simulink model "APF_Path_Planning_2023a"  (R2023a)
settings: Solver=ode4  StartTime=0.0  StopTime=tsim  FixedStep=baseRate  RelTol=1e-6  AbsTol=1e-6
values from neighbouring files (symbols this model uses):
  A = [0 0 0 1 0 0 ... (first row only)    [CTL.m]
  a = 25.028    [CTL.m]
  a1 = gain_matrix(1,1)    [CTL.m]
  alpha_m = 0.1    [CTL.m]
  alphap = 1    [CTL.m]
  alphat = 1.1    [CTL.m]
  Am = [0 0 1 0; 0 0 0 1; -wn^2 0 -2*zeta*wn 0; 0 -wn^2 0 -2*zeta*wn]    [CTL.m]
  b = gain_matrix(1,2)    [CTL.m]
  Bm = [0 0; 0 0; -wn^2 0; 0 -wn^2]    [CTL.m]
  c = gain_matrix(2,1)    [CTL.m]
  Cm = [alpha_m 0 0 0; 0 alpha_m 0 0; 0 0 1 0; 0 0 0 1]    [CTL.m]
  d = gain_matrix(2,2)    [CTL.m]
  Dm = zeros(4,2)    [CTL.m]
  epsilon = F_max/2    (= 0.11)    [CTL.m]
  F_max = 0.22    [CTL.m]
  Hz = 0.01    [CTL.m]
  J = IRED    [CTL.m]
  k = lqr(A,B1,Q,R)    [CTL.m]
  k1 = 5    [CTL.m]
  k1t = 2    [CTL.m]
  k2 = 28    [CTL.m]
  k2t = 16    [CTL.m]
  k_1_0 = 3.5    [CTL.m]
  k_1_t_0 = 1    [CTL.m]
  k_2_0 = 28    [CTL.m]
  k_2_t_0 = 1    [CTL.m]
  Kd_t = 9.5    [CTL.m]
  Kd_x = 28    [CTL.m]
  Kd_y = Kd_x    (= 28)    [CTL.m]
  Kp_t = 1    [CTL.m]
  Kp_x = 3.5    [CTL.m]
  Kp_y = Kp_x    (= 3.5)    [CTL.m]
  lambda1 = 0.4    [CTL.m]
  lambda12 = 0.4    [CTL.m]
  lambda12_t = 0.05    [CTL.m]
  lambda1_t = 0.05    [CTL.m]
  lambda2 = 0.4    [CTL.m]
  lambda2_t = 0.05    [CTL.m]
  m = mRED    [CTL.m]
  p = 0.4    [CTL.m]
  p_t = 0.05    [CTL.m]
  Q = [w 0 0 0 0 0 ... (first row only)    [CTL.m]
  R = [r 0 0 ... (first row only)    [CTL.m]
  Red_Rate = 0.025    [CTL.m]
  T_max = 0.0235    [CTL.m]
  Time_Look = 25    [CTL.m]
  xm_0 = [RED_ini(1,1:2),0,0]    [CTL.m]
undefined symbols (not defined in the file or in its folder): a2, a3, adadelta_epsilon, adadelta_gamma, adagrad_epsilon, adagrad_eta, adam_beta_1, adam_beta_2, adam_epsilon, adam_eta, adamax_beta_1, adamax_beta_2, adamax_eta, alpha, Att_Mode, b0, b1, b2, b3, baseRate, beta, Binv, BLACK_end, BLACK_ini, BLUE_end, BLUE_ini, DiscIntNeverNeededParam, drop_states_ARM, drop_states_BLACK, drop_states_BLUE, drop_states_RED, dt, end_time_black, end_time_blue, F_Black_X_nominal, F_Black_Y_nominal, F_Blue_X_nominal, F_Blue_Y_nominal, F_red_X_nominal, F_red_Y_nominal, F_thrusters_BLACK, F_thrusters_BLUE, F_thrusters_RED, Gamma1_el, Gamma1_sh, Gamma1_wr, Gamma2_el, Gamma2_sh, Gamma2_wr, Gamma3_el, Gamma3_sh, Gamma3_wr, Gamma4_el, Gamma4_sh, Gamma4_wr, Gamma5_el, Gamma5_sh, Gamma5_wr, Gamma6_el, Gamma6_sh ... (+98)
libraries: nvidiaSharedBlocks x10, MainLibrary x4, dspsigops x4, simulink x2, etargetslib x1
(part 11 of 13)

== system APF_Path_Planning_2023a/Phase #3: Experiment/Change RED Behavior/Sub-Phase #4/RED+ARM/Simulated Position Controller/Custom Discrete PD (Elbow)/x_dot -> x2 ==
  note: dy/dt ~= (y2-y1)/deltaT
  y(t) : Inport
  Delay1 : Delay  DelayLength=1  InitialConditionSource=Input port
      settings: InputPortMap=u0,p4
  Hold this value : Subsystem  TreatAsAtomicUnit=on
  Sum6 : Sum  Inputs=-+|
  divide by delta T : Gain  Gain=1/baseRate
  "if we went through a \"step\"" : If  IfExpression=u1 ~= 0  ShowElse=off
  dy(t)/dt : Outport  VectorParamsAs1DForOutWhenUnconnected=off
  wires:
  divide by delta T/1 -> dy(t)/dt/1
  Delay1/1 -> Sum6/1
  "if we went through a \"step\""/1 -> Hold this value/Action
  Hold this value/1(Out1) -> divide by delta T/1
  Sum6/1 -> "if we went through a \"step\""/1, Hold this value/1(In1)
  y(t)/1 -> Sum6/2, Delay1/2, Delay1/1

== system APF_Path_Planning_2023a/Phase #3: Experiment/Change RED Behavior/Sub-Phase #4/RED+ARM/Simulated Position Controller/Custom Discrete PD (Shoulder)/x_dot -> x2 ==
  note: dy/dt ~= (y2-y1)/deltaT
  y(t) : Inport
  Delay1 : Delay  DelayLength=1  InitialConditionSource=Input port
      settings: InputPortMap=u0,p4
  Hold this value : Subsystem  TreatAsAtomicUnit=on
  Sum6 : Sum  Inputs=-+|
  divide by delta T : Gain  Gain=1/baseRate
  "if we went through a \"step\"" : If  IfExpression=u1 ~= 0  ShowElse=off
  dy(t)/dt : Outport  VectorParamsAs1DForOutWhenUnconnected=off
  wires:
  divide by delta T/1 -> dy(t)/dt/1
  Delay1/1 -> Sum6/1
  "if we went through a \"step\""/1 -> Hold this value/Action
  Hold this value/1(Out1) -> divide by delta T/1
  Sum6/1 -> "if we went through a \"step\""/1, Hold this value/1(In1)
  y(t)/1 -> Sum6/2, Delay1/2, Delay1/1

== system APF_Path_Planning_2023a/Phase #3: Experiment/Change RED Behavior/Sub-Phase #4/RED+ARM/Simulated Position Controller/Custom Discrete PD (Wrist)/x_dot -> x2 ==
  note: dy/dt ~= (y2-y1)/deltaT
  y(t) : Inport
  Delay1 : Delay  DelayLength=1  InitialConditionSource=Input port
      settings: InputPortMap=u0,p4
  Hold this value : Subsystem  TreatAsAtomicUnit=on
  Sum6 : Sum  Inputs=-+|
  divide by delta T : Gain  Gain=1/baseRate
  "if we went through a \"step\"" : If  IfExpression=u1 ~= 0  ShowElse=off
  dy(t)/dt : Outport  VectorParamsAs1DForOutWhenUnconnected=off
  wires:
  divide by delta T/1 -> dy(t)/dt/1
  Delay1/1 -> Sum6/1
  "if we went through a \"step\""/1 -> Hold this value/Action
  Hold this value/1(Out1) -> divide by delta T/1
  Sum6/1 -> "if we went through a \"step\""/1, Hold this value/1(In1)
  y(t)/1 -> Sum6/2, Delay1/2, Delay1/1

== system APF_Path_Planning_2023a/Phase #4: Return Home/Change RED Behavior/RED+ARM/Simulated Position Controller/Custom Discrete PD (Elbow)/x_dot -> x2/Hold this value ==
  In1 : Inport
  Action Port : ActionPort  ActionPortLabel=if(u1 ~= 0)
  Out1 : Outport  VectorParamsAs1DForOutWhenUnconnected=off
  wires:
  In1/1 -> Out1/1

== system APF_Path_Planning_2023a/Phase #4: Return Home/Change RED Behavior/RED+ARM/Simulated Position Controller/Custom Discrete PD (Shoulder)/x_dot -> x2/Hold this value ==
  In1 : Inport
  Action Port : ActionPort  ActionPortLabel=if(u1 ~= 0)
  Out1 : Outport  VectorParamsAs1DForOutWhenUnconnected=off
  wires:
  In1/1 -> Out1/1

== system APF_Path_Planning_2023a/Phase #4: Return Home/Change RED Behavior/RED+ARM/Simulated Position Controller/Custom Discrete PD (Wrist)/x_dot -> x2/Hold this value ==
  In1 : Inport
  Action Port : ActionPort  ActionPortLabel=if(u1 ~= 0)
  Out1 : Outport  VectorParamsAs1DForOutWhenUnconnected=off
  wires:
  In1/1 -> Out1/1

== system APF_Path_Planning_2023a/Phase #5: Hold Home/Change RED Behavior/RED+ARM/Simulated Position Controller/Custom Discrete PD (Elbow)/x_dot -> x2/Hold this value ==
  In1 : Inport
  Action Port : ActionPort  ActionPortLabel=if(u1 ~= 0)
  Out1 : Outport  VectorParamsAs1DForOutWhenUnconnected=off
  wires:
  In1/1 -> Out1/1

== system APF_Path_Planning_2023a/Phase #5: Hold Home/Change RED Behavior/RED+ARM/Simulated Position Controller/Custom Discrete PD (Shoulder)/x_dot -> x2/Hold this value ==
  In1 : Inport
  Action Port : ActionPort  ActionPortLabel=if(u1 ~= 0)
  Out1 : Outport  VectorParamsAs1DForOutWhenUnconnected=off
  wires:
  In1/1 -> Out1/1

== system APF_Path_Planning_2023a/Phase #5: Hold Home/Change RED Behavior/RED+ARM/Simulated Position Controller/Custom Discrete PD (Wrist)/x_dot -> x2/Hold this value ==
  In1 : Inport
  Action Port : ActionPort  ActionPortLabel=if(u1 ~= 0)
  Out1 : Outport  VectorParamsAs1DForOutWhenUnconnected=off
  wires:
  In1/1 -> Out1/1

== system APF_Path_Planning_2023a/Phase #3: Experiment/Change RED Behavior/Sub-Phase #1/RED+ARM/Simulated Position Controller/Custom Discrete PD (Elbow)/x_dot -> x2/Hold this value ==
  In1 : Inport
  Action Port : ActionPort  ActionPortLabel=if(u1 ~= 0)
  Out1 : Outport  VectorParamsAs1DForOutWhenUnconnected=off
  wires:
  In1/1 -> Out1/1

== system APF_Path_Planning_2023a/Phase #3: Experiment/Change RED Behavior/Sub-Phase #1/RED+ARM/Simulated Position Controller/Custom Discrete PD (Shoulder)/x_dot -> x2/Hold this value ==
  In1 : Inport
  Action Port : ActionPort  ActionPortLabel=if(u1 ~= 0)
  Out1 : Outport  VectorParamsAs1DForOutWhenUnconnected=off
  wires:
  In1/1 -> Out1/1

== system APF_Path_Planning_2023a/Phase #3: Experiment/Change RED Behavior/Sub-Phase #1/RED+ARM/Simulated Position Controller/Custom Discrete PD (Wrist)/x_dot -> x2/Hold this value ==
  In1 : Inport
  Action Port : ActionPort  ActionPortLabel=if(u1 ~= 0)
  Out1 : Outport  VectorParamsAs1DForOutWhenUnconnected=off
  wires:
  In1/1 -> Out1/1

== system APF_Path_Planning_2023a/Phase #3: Experiment/Change RED Behavior/Sub-Phase #2 /RED+ARM/Simulated Position Controller/Custom Discrete PD (Elbow)/x_dot -> x2/Hold this value ==
  In1 : Inport
  Action Port : ActionPort  ActionPortLabel=if(u1 ~= 0)
  Out1 : Outport  VectorParamsAs1DForOutWhenUnconnected=off
  wires:
  In1/1 -> Out1/1

== system APF_Path_Planning_2023a/Phase #3: Experiment/Change RED Behavior/Sub-Phase #2 /RED+ARM/Simulated Position Controller/Custom Discrete PD (Shoulder)/x_dot -> x2/Hold this value ==
  In1 : Inport
  Action Port : ActionPort  ActionPortLabel=if(u1 ~= 0)
  Out1 : Outport  VectorParamsAs1DForOutWhenUnconnected=off
  wires:
  In1/1 -> Out1/1

== system APF_Path_Planning_2023a/Phase #3: Experiment/Change RED Behavior/Sub-Phase #2 /RED+ARM/Simulated Position Controller/Custom Discrete PD (Wrist)/x_dot -> x2/Hold this value ==
  In1 : Inport
  Action Port : ActionPort  ActionPortLabel=if(u1 ~= 0)
  Out1 : Outport  VectorParamsAs1DForOutWhenUnconnected=off
  wires:
  In1/1 -> Out1/1

== system APF_Path_Planning_2023a/Phase #3: Experiment/Change RED Behavior/Sub-Phase #3 /RED+ARM/Simulated Position Controller/Custom Discrete PD (Elbow)/x_dot -> x2/Hold this value ==
  In1 : Inport
  Action Port : ActionPort  ActionPortLabel=if(u1 ~= 0)
  Out1 : Outport  VectorParamsAs1DForOutWhenUnconnected=off
  wires:
  In1/1 -> Out1/1

== system APF_Path_Planning_2023a/Phase #3: Experiment/Change RED Behavior/Sub-Phase #3 /RED+ARM/Simulated Position Controller/Custom Discrete PD (Shoulder)/x_dot -> x2/Hold this value ==
  In1 : Inport
  Action Port : ActionPort  ActionPortLabel=if(u1 ~= 0)
  Out1 : Outport  VectorParamsAs1DForOutWhenUnconnected=off
  wires:
  In1/1 -> Out1/1

== system APF_Path_Planning_2023a/Phase #3: Experiment/Change RED Behavior/Sub-Phase #3 /RED+ARM/Simulated Position Controller/Custom Discrete PD (Wrist)/x_dot -> x2/Hold this value ==
  In1 : Inport
  Action Port : ActionPort  ActionPortLabel=if(u1 ~= 0)
  Out1 : Outport  VectorParamsAs1DForOutWhenUnconnected=off
  wires:
  In1/1 -> Out1/1

== system APF_Path_Planning_2023a/Phase #3: Experiment/Change RED Behavior/Sub-Phase #4/CTL/Subsystem1/Custom Discrete PD (Attitude)/x_dot -> x2/Hold this value ==
  In1 : Inport
  Action Port : ActionPort  ActionPortLabel=if(u1 ~= 0)
  Out1 : Outport  VectorParamsAs1DForOutWhenUnconnected=off
  wires:
  In1/1 -> Out1/1

== system APF_Path_Planning_2023a/Phase #3: Experiment/Change RED Behavior/Sub-Phase #4/GDC/APF/GDC/Subsystem1/AdaDelta ==
  state_red : Inport
  phi_tot_grad : Inport  Port=2
  Delay : Delay  DelayLength=1  InitialCondition=[0;0;0]
  Delay1 : Delay  DelayLength=1  InitialCondition=[0;0;0]
  MATLAB Function1 : MATLAB Function  TreatAsAtomicUnit=on
  path : Outport
  wires:
  MATLAB Function1/2(Eg) -> Delay/1
  Delay/1 -> MATLAB Function1/3(Eg_old)
  MATLAB Function1/3(Etheta) -> Delay1/1
  Delay1/1 -> MATLAB Function1/4(Etheta_old)
  phi_tot_grad/1 -> MATLAB Function1/2(phi_tot_grad)
  state_red/1 -> MATLAB Function1/1(state_red)
  MATLAB Function1/1(path) -> path/1

== system APF_Path_Planning_2023a/Phase #3: Experiment/Change RED Behavior/Sub-Phase #4/GDC/APF/GDC/Subsystem1/AdaGrad ==
  phit_tot_grad : Inport
  state_red : Inport  Port=2
  Delay3 : Delay  DelayLength=1
  MATLAB Function1 : MATLAB Function  TreatAsAtomicUnit=on
  path : Outport
  wires:
  state_red/1 -> MATLAB Function1/1(state_red)
  Delay3/1 -> MATLAB Function1/3(Gt_old)
  MATLAB Function1/1(path) -> path/1
  phit_tot_grad/1 -> MATLAB Function1/2(phi_tot_grad)
  MATLAB Function1/2(Gt) -> Delay3/1

== system APF_Path_Planning_2023a/Phase #3: Experiment/Change RED Behavior/Sub-Phase #4/GDC/APF/GDC/Subsystem1/AdaMax ==
  phit_tot_grad : Inport
  state_red : Inport  Port=2
  Clock : Clock
  Constant : Constant  Value=Phase2_End
  Delay1 : Delay  DelayLength=1
  Delay3 : Delay  DelayLength=1
  MATLAB Function1 : MATLAB Function  TreatAsAtomicUnit=on
  Sum : Sum  Inputs=|+-
  path : Outport
  wires:
  Delay1/1 -> MATLAB Function1/4(v_old)
  MATLAB Function1/3(v) -> Delay1/1
  MATLAB Function1/2(m) -> Delay3/1
  Delay3/1 -> MATLAB Function1/3(m_old)
  state_red/1 -> MATLAB Function1/1(state_red)
  phit_tot_grad/1 -> MATLAB Function1/2(phi_tot_grad)
  MATLAB Function1/1(path) -> path/1
  Clock/1 -> Sum/1
  Sum/1 -> MATLAB Function1/5(time)
  Constant/1 -> Sum/2

== system APF_Path_Planning_2023a/Phase #3: Experiment/Change RED Behavior/Sub-Phase #4/GDC/APF/GDC/Subsystem1/Adam ==
  phit_tot_grad : Inport
  state_red : Inport  Port=2
  Clock : Clock
  Delay1 : Delay  DelayLength=1
  Delay3 : Delay  DelayLength=1
  MATLAB Function1 : MATLAB Function  TreatAsAtomicUnit=on
  path : Outport
  wires:
  MATLAB Function1/1(path) -> path/1
  phit_tot_grad/1 -> MATLAB Function1/2(phi_tot_grad)
  state_red/1 -> MATLAB Function1/1(state_red)
  Delay3/1 -> MATLAB Function1/3(m_old)
  MATLAB Function1/2(m) -> Delay3/1
  Clock/1 -> MATLAB Function1/5(time)
  MATLAB Function1/3(v) -> Delay1/1
  Delay1/1 -> MATLAB Function1/4(v_old)

== system APF_Path_Planning_2023a/Phase #3: Experiment/Change RED Behavior/Sub-Phase #4/GDC/APF/GDC/Subsystem1/Gradient Descent ==
  state_red : Inport
  phi_tot_grad : Inport  Port=2
  Batch : MATLAB Function  TreatAsAtomicUnit=on
  path : Outport
  wires:
  Batch/1(path) -> path/1
  phi_tot_grad/1 -> Batch/2(phi_tot_grad)
  state_red/1 -> Batch/1(state_red)

== system APF_Path_Planning_2023a/Phase #3: Experiment/Change RED Behavior/Sub-Phase #4/GDC/APF/GDC/Subsystem1/Momentum ==
  phi_tot_grad : Inport
  state_red : Inport  Port=2
  Constant : Constant  Value=[0;0;0]
  Delay : Delay  DelayLength=1
  Momentum : MATLAB Function  TreatAsAtomicUnit=on
  Sum3 : Sum  Inputs=|++
  path : Outport
  wires:
  Constant/1 -> Sum3/2
  Delay/1 -> Momentum/3(v_prev)
  Momentum/1(path) -> path/1
  Momentum/2(v) -> Sum3/1
  phi_tot_grad/1 -> Momentum/2(phi_tot_grad)
  Sum3/1 -> Delay/1
  state_red/1 -> Momentum/1(state_red)

== system APF_Path_Planning_2023a/Phase #3: Experiment/Change RED Behavior/Sub-Phase #4/GDC/APF/GDC/Subsystem1/Nesterov ==
  state_red : Inport
  state_black : Inport  Port=2
  state_blue : Inport  Port=3
  Constant1 : Constant  Value=[0;0;0]
  Delay : Delay  DelayLength=1
  MATLAB Function1 : MATLAB Function  TreatAsAtomicUnit=on
  Sum : Sum  Inputs=|++
  path : Outport
  wires:
  MATLAB Function1/2(v) -> Sum/1
  Delay/1 -> MATLAB Function1/2(v_prev)
  Constant1/1 -> Sum/2
  MATLAB Function1/1(path) -> path/1
  Sum/1 -> Delay/1
  state_red/1 -> MATLAB Function1/1(state_red)
  state_black/1 -> MATLAB Function1/3(state_black)
  state_blue/1 -> MATLAB Function1/4(state_blue)

== system APF_Path_Planning_2023a/Phase #3: Experiment/Change RED Behavior/Sub-Phase #4/GDC/APF/GDC/Subsystem1/RMSProp ==
  phit_tot_grad : Inport
  state_red : Inport  Port=2
  Delay3 : Delay  DelayLength=1
  MATLAB Function1 : MATLAB Function  TreatAsAtomicUnit=on
  path : Outport
  wires:
  MATLAB Function1/2(Eg) -> Delay3/1
  Delay3/1 -> MATLAB Function1/3(Eg_old)
  state_red/1 -> MATLAB Function1/1(state_red)
  phit_tot_grad/1 -> MATLAB Function1/2(phi_tot_grad)
  MATLAB Function1/1(path) -> path/1

== system APF_Path_Planning_2023a/Phase #3: Experiment/Change RED Behavior/Sub-Phase #4/RED+ARM/Simulated Position Controller/Custom Discrete PD (Elbow)/x_dot -> x2/Hold this value ==
  In1 : Inport
  Action Port : ActionPort  ActionPortLabel=if(u1 ~= 0)
  Out1 : Outport  VectorParamsAs1DForOutWhenUnconnected=off
  wires:
  In1/1 -> Out1/1

== system APF_Path_Planning_2023a/Phase #3: Experiment/Change RED Behavior/Sub-Phase #4/RED+ARM/Simulated Position Controller/Custom Discrete PD (Shoulder)/x_dot -> x2/Hold this value ==
  In1 : Inport
  Action Port : ActionPort  ActionPortLabel=if(u1 ~= 0)
  Out1 : Outport  VectorParamsAs1DForOutWhenUnconnected=off
  wires:
  In1/1 -> Out1/1

== system APF_Path_Planning_2023a/Phase #3: Experiment/Change RED Behavior/Sub-Phase #4/RED+ARM/Simulated Position Controller/Custom Discrete PD (Wrist)/x_dot -> x2/Hold this value ==
  In1 : Inport
  Action Port : ActionPort  ActionPortLabel=if(u1 ~= 0)
  Out1 : Outport  VectorParamsAs1DForOutWhenUnconnected=off
  wires:
  In1/1 -> Out1/1

== matlab function APF_Path_Planning_2023a/Phase #3: Experiment/Change RED Behavior/Sub-Phase #2 /MATLAB Function ==
  data: t input; x output; xLength parameter
function x = fcn(t, xLength)

x = 0.9*cos((0.03490659)*t) + xLength/2;

end

== matlab function APF_Path_Planning_2023a/Phase #3: Experiment/Change RED Behavior/Sub-Phase #2 /MATLAB Function1 ==
  data: t input; y output; yLength parameter
function y = fcn(t, yLength)

y = 0.85*sin((0.03490659)*t) + yLength/2;

end

== matlab function APF_Path_Planning_2023a/Phase #3: Experiment/Change RED Behavior/Sub-Phase #3 /Hough Control/MATLAB Function2 ==
  data: Oy output; z input; Ox output
function [Oy, Ox]   = C3( z )
%C3 gives the rotation matrix about the z-axis for an angle 'z'
%   z - the angle about the z-axis which you rotate
%   A - the rotation matrix

Ox = [cos(z) sin(z); -sin(z) cos(z)]*[1;0];
Oy = [cos(z) sin(z); -sin(z) cos(z)]*[0;1];
end

== matlab function APF_Path_Planning_2023a/Phase #3: Experiment/Change RED Behavior/Sub-Phase #3 /Hough Control/MATLAB Function3 ==
  data: z input; Ox output
function Ox    = C3( z )
%C3 gives the rotation matrix about the z-axis for an angle 'z'
%   z - the angle about the z-axis which you rotate
%   A - the rotation matrix

Ox = [cos(z) sin(z); -sin(z) cos(z)]*[1;0];
end

== matlab function APF_Path_Planning_2023a/Phase #3: Experiment/Change RED Behavior/Sub-Phase #3 /Hough Control/MATLAB Function4 ==
  data: Oy input; e_out output; e_in input
function e_out = fcn(Oy, e_in)

a = sign(Oy'*e_in);
e_out = -a*norm(e_in);

== matlab function APF_Path_Planning_2023a/Phase #3: Experiment/Change RED Behavior/Sub-Phase #3 /MATLAB Function ==
  data: t input; x output; xLength parameter
function x = fcn(t, xLength)

x = 0.9*cos((0.03490659)*t) + xLength/2;

end

== matlab function APF_Path_Planning_2023a/Phase #3: Experiment/Change RED Behavior/Sub-Phase #3 /MATLAB Function1 ==
  data: t input; y output; yLength parameter
function y = fcn(t, yLength)

y = 0.85*sin((0.03490659)*t) + yLength/2;

end

== matlab function APF_Path_Planning_2023a/Phase #3: Experiment/Change BLACK Behavior/Sub-Phase #3 /BLACK_Rz Desired/Wrap1/MATLAB Function ==
  data: u input; wrappedAngle output
function wrappedAngle = wrapAngle(u)

wrappedAngle = atan2(sin(u),cos(u));

end

== matlab function APF_Path_Planning_2023a/Phase #3: Experiment/Change BLACK Behavior/Sub-Phase #3 /Hough Control/MATLAB Function2 ==
  data: Oy output; z input; Ox output
function [Oy, Ox]   = C3( z )
%C3 gives the rotation matrix about the z-axis for an angle 'z'
%   z - the angle about the z-axis which you rotate
%   A - the rotation matrix

Ox = [cos(z) sin(z); -sin(z) cos(z)]*[1;0];
Oy = [cos(z) sin(z); -sin(z) cos(z)]*[0;1];
end

== matlab function APF_Path_Planning_2023a/Phase #5: Hold Home/Change BLACK Behavior/Hough Control/MATLAB Function3 ==
  data: z input; Ox output
function Ox    = C3( z )
%C3 gives the rotation matrix about the z-axis for an angle 'z'
%   z - the angle about the z-axis which you rotate
%   A - the rotation matrix

Ox = [cos(z) sin(z); -sin(z) cos(z)]*[1;0];
end

== matlab function APF_Path_Planning_2023a/Phase #3: Experiment/Change BLACK Behavior/Sub-Phase #3 /Hough Control/MATLAB Function3 ==
  data: z input; Ox output
function Ox    = C3( z )
%C3 gives the rotation matrix about the z-axis for an angle 'z'
%   z - the angle about the z-axis which you rotate
%   A - the rotation matrix

Ox = [cos(z) sin(z); -sin(z) cos(z)]*[1;0];
end

== matlab function APF_Path_Planning_2023a/Phase #3: Experiment/Change BLUE Behavior/Sub-Phase #1/MATLAB Function2 ==
  data: t input; x output; xLength parameter
function x = fcn(t, xLength)

x = -0.85*cos((0.03490659)*t) + xLength/2;

end

== matlab function APF_Path_Planning_2023a/Phase #3: Experiment/Change BLACK Behavior/Sub-Phase #1/Hough Control/MATLAB Function4 ==
  data: Oy input; e_out output; e_in input
function e_out = fcn(Oy, e_in)

a = sign(Oy'*e_in);
e_out = -a*norm(e_in);

== matlab function APF_Path_Planning_2023a/Phase #3: Experiment/Change BLUE Behavior/Sub-Phase #1/MATLAB Function3 ==
  data: t input; y output; yLength parameter
function y = fcn(t, yLength)

y = -0.85*sin((0.03490659)*t) + yLength/2;

end

== matlab function APF_Path_Planning_2023a/Phase #3: Experiment/Change RED Behavior/Sub-Phase #4/CTL/If Action Subsystem/Homo/MATLAB Function3 ==
  data: q2 input; u output; k2 parameter; alphap parameter
function u = fcn(q2,k2, alphap)

u = k2*sign(q2)*(abs(q2)^alphap);

== matlab function APF_Path_Planning_2023a/Phase #3: Experiment/Change RED Behavior/Sub-Phase #4/GDC/APF/Looking Angle ==
  data: state_black input; state_red input; theta_desired output; r_off parameter
function theta_desired = fcn(state_black, state_red, r_off)

p_l = [state_black(1) + r_off*cos(state_black(3));
       state_black(2) + r_off*sin(state_black(3))];

p_c_1 = state_red(1:2);
r_cl = p_c_1 - p_l;

r_cl_x = r_cl(1);
r_cl_y = r_cl(2);

theta_desired = angle(r_cl_x + j*r_cl_y) + pi;

== matlab function APF_Path_Planning_2023a/Phase #3: Experiment/Change RED Behavior/Sub-Phase #4/CTL/Hough Control/MATLAB Function2 ==
  data: Oy output; z input; Ox output
function [Oy, Ox]   = C3( z )
%C3 gives the rotation matrix about the z-axis for an angle 'z'
%   z - the angle about the z-axis which you rotate
%   A - the rotation matrix

Ox = [cos(z) sin(z); -sin(z) cos(z)]*[1;0];
Oy = [cos(z) sin(z); -sin(z) cos(z)]*[0;1];
end

== matlab function APF_Path_Planning_2023a/PhaseSpace Camera Code/Use Hardware to Obtain States/MATLAB Function ==
  data: StartClock output; RedReceiving input; BlackReceiving input; BlueReceiving input; platformSelection parameter
function StartClock = CheckForSync(RedReceiving, BlackReceiving, BlueReceiving, platformSelection)
        
    StartClock = 0;
    
    if (platformSelection == 1)
        
        if RedReceiving == 1

            StartClock = 1;

        else

            StartClock = 0;

        end
        
    elseif (platformSelection == 2)
        
        if BlackReceiving == 1

            StartClock = 1;

        else

            StartClock = 0;

        end  
        
    elseif (platformSelection == 3)
        
        if RedReceiving == 1 && BlackReceiving == 1

            StartClock = 1;

        else

            StartClock = 0;

        end    
        
    elseif (platformSelection == 4)
        
        if RedReceiving == 1 && BlackReceiving == 1

            StartClock = 1;

        else

            StartClock = 0;

        end
        
    elseif (platformSelection == 5)
        
        if RedReceiving == 1

            StartClock = 1;

        else

            StartClock = 0;

        end
        
    elseif (platformSelection == 6)
        
        if BlueReceiving == 1

            StartClock = 1;

        else

            StartClock = 0;

        end
        
    elseif (platformSelection == 7)
        
        if RedReceiving == 1 && BlueReceiving == 1

            StartClock = 1;

        else

            StartClock = 0;

        end
        
    elseif (platformSelection == 8)
        
        if RedReceiving == 1 && BlackReceiving == 1 && BlueReceiving == 1

            StartClock = 1;

        else

            StartClock = 0;

        end
        
    elseif (platformSelection == 9)
        
        if BlackReceiving == 1 && BlueReceiving == 1

            StartClock = 1;

        else

            StartClock = 0;

        end
                           
    elseif (platformSelection == 10)
        
        if RedReceiving == 1 && BlueReceiving == 1

            StartClock = 1;

        else

            StartClock = 0;

        end
        
    elseif (platformSelection == 11)
        
        if RedReceiving == 1 && BlackReceiving == 1 && BlueReceiving == 1

            StartClock = 1;

        else

            StartClock = 0;

        end
        
    end



end

== matlab function APF_Path_Planning_2023a/Phase #5: Hold Home/Change BLACK Behavior/Hough Control/MATLAB Function4 ==
  data: Oy input; e_out output; e_in input
function e_out = fcn(Oy, e_in)

a = sign(Oy'*e_in);
e_out = -a*norm(e_in);

== matlab function APF_Path_Planning_2023a/Phase #3: Experiment/Change RED Behavior/Sub-Phase #4/CTL/Hough Control/MATLAB Function3 ==
  data: z input; Ox output
function Ox    = C3( z )
%C3 gives the rotation matrix about the z-axis for an angle 'z'
%   z - the angle about the z-axis which you rotate
%   A - the rotation matrix

Ox = [cos(z) sin(z); -sin(z) cos(z)]*[1;0];
end

== matlab function APF_Path_Planning_2023a/Phase #3: Experiment/Change RED Behavior/Sub-Phase #4/CTL/If Action Subsystem/DAC Controller1/Fx Gain Derivatives ==
  data: e_xdot input; k2_dot output; e_x input; k1_dot output; lambda1 parameter; lambda2 parameter; lambda12 parameter; p parameter
function [k2_dot, k1_dot]= fcn(e_xdot, e_x, lambda1, lambda2, lambda12, p)

k1_dot = -lambda1*p*e_x^2-(lambda1+p*lambda12)*e_x*e_xdot-lambda12*e_xdot^2;
k2_dot = -lambda12*p*e_x^2-(lambda12+p*lambda2)*e_x*e_xdot-lambda2*e_xdot^2;

== matlab function APF_Path_Planning_2023a/Phase #3: Experiment/Change RED Behavior/Sub-Phase #4/CTL/Hough Control/MATLAB Function4 ==
  data: Oy input; e_out output; e_in input
function e_out = fcn(Oy, e_in)

a = sign(Oy'*e_in);
e_out = -a*norm(e_in);

== matlab function APF_Path_Planning_2023a/Phase #3: Experiment/Change RED Behavior/Sub-Phase #1/RED_Rz Desired/Wrap/MATLAB Function ==
  data: u input; wrappedAngle output
function wrappedAngle = wrapAngle(u)

wrappedAngle = atan2(sin(u),cos(u));

end

== matlab function APF_Path_Planning_2023a/Phase #3: Experiment/Change RED Behavior/Sub-Phase #4/BLACK/Ryan's Transform ==
  data: Measurments input; Black_Measurments_table_ref output; Red_States input; delta parameter
function Black_Measurments_table_ref = RelitivetoTable(Measurments,Red_States,delta)
 Measurments(1) = Measurments(1)/100;
 Measurments(2) = Measurments(2)/100;
 Measurments(3) = Measurments(3)*pi/180;

%% This code is very scuffed, so I added lots of notes, feel free to change this
%% Size check
if size(Red_States,1) == 6 || size(Red_States,2) == 6
    Red_States = Red_States(1:3);
elseif size(Red_States,1) == 3 || size(Red_States,2) == 3
    % Nothin
else
    disp('Error with demensions of Red_States')
    disp('Please use 3 or 6 states')
    disp(':(')
end

if size(Measurments,1) == 3 || size(Measurments,2) == 3
    % Nothin
else
    disp('Error with demensions of Measurments')
    disp('VIS only gives 3 states, please only use 3 states')
    disp(':(')
end
Red_States(3) = mod(Red_States(3) + pi, 2*pi) - pi;

%% Rotation matrix scuffed (accounts for the location change of the docking cone) + Camera Offset of 3 deg
     c3 = [sin(Red_States(3) + delta*pi/180),  cos(Red_States(3) + delta*pi/180), 0;
          cos(Red_States(3) + delta*pi/180), -sin(Red_States(3) + delta*pi/180), 0;
          0,                     0,                    1];

%% Measurments in table ref frame
    Black_Measurments_table_ref = c3*Measurments;

%% Vector addition
    Black_Measurments_table_ref(1) = Black_Measurments_table_ref(1) + Red_States(1); 
    Black_Measurments_table_ref(2) =  -1*Black_Measurments_table_ref(2) + Red_States(2); % Negative Y value accounting for "Left Hand Rule"

%% Angle addition
    Black_Measurments_table_ref(3) = Measurments(3) + Red_States(3) - pi/2; % Pi/2 for the docking cone location offset from Phase Space

%% Wrapping Angle from -pi to pi
% Dont ask me why, its consistant with the SPOT inport from phasespace
% Dont belive me, look at this, angular velocity is being unwrapped, therefor, angle must be wrapped
% APF_Path_Planning_2023a/PhaseSpace Camera Code/Use Hardware to Obtain States
    % Black_Measurments_table_ref(3) = mod(Black_Measurments_table_ref(3) + pi, 2*pi) - pi;
end

== matlab function APF_Path_Planning_2023a/Phase #3: Experiment/Change RED Behavior/Sub-Phase #4/BLACK/UKF_New/MATLAB Function2 ==
  data: no_IC output; Rejection output; Measurments input; Force input; States_k1 input; N_Rejectk1 input; States output; N_Rejectk output; P_K output; P_K1 input; lamda parameter; J parameter; m parameter; dt parameter; Q parameter; alpha parameter; beta parameter; H parameter; R parameter; thresh parameter; method parameter
function [no_IC,Rejection,States,N_Rejectk,P_K] = UKF(Measurments,Force,States_k1,N_Rejectk1,P_K1, lamda, J, m, dt, Q, alpha, beta, H, R,thresh,method)
%% Block diagram got messy so i put it all in one block
if isempty(Force)
    Force = [0;0;0];
end

%% Inital position
if all(States_k1 == 0) || anynan(States_k1)
    if anynan(Measurments)
        States = NaN(6,1);
        no_IC = 1;
        P_K = P_K1;
    else
        States = [Measurments;zeros(3,1)];
        no_IC = 0;
        P_K = P_K1;
    end
else
    no_IC = 0;

    X_Cal = fcn1(States_k1,P_K1,lamda,method);
    
    X_Cal_k1 = fcn2(Force,X_Cal,J,m,dt);
    
    [w_m,w_c,X_tilda_k,P_K1] = fcn3(X_Cal_k1,lamda, Q, alpha, beta);
    
    [Z_Bar,Z_Cal] = fcn4(X_Cal_k1, w_m,H);
    
    [P_xz_k,P_z_k] = fcn5(Z_Bar,Z_Cal,w_c,X_tilda_k,X_Cal,R);
    
    K_k = fcn6(P_xz_k,P_z_k);
    
    Z_k = fcn7(Measurments);

    thresh_dynamic = Dynamic_Threshold(N_Rejectk1,thresh);
    
    Reject = fcn8(Z_k,Z_Bar,P_z_k,thresh_dynamic);

    N_Rejectk = Was_rejected(Reject,N_Rejectk1);
    
    States = fcn9(Z_k,Reject,X_tilda_k,Z_Bar,K_k);
    
    P_K = fcn10(P_K1,P_z_k,K_k,Reject);
end
end

function X_Cal = fcn1(x_tilda_k,P_k,lamda,method)
%% Calculate size of sigma var
sz = 6;
N = 2*sz + 1;
X_Cal = zeros(sz,N);

%% Calculate initial sigma point
X_Cal(:,1) = x_tilda_k;

%% Calculate sigma distance
sigma = (6 + lamda)*P_k;
sigma = Cholesky_Decomposition(sigma,method);

%% Calculate Sigma Points
% Positive points
for i = 2:1:((N-1)/2) + 1
    fill = zeros(size(x_tilda_k));
    fill(i-1,1) = sigma(i-1,i-1);
    X_Cal(:,i) = x_tilda_k + fill;
end
% Negative Points
j = 1;
for i = N + 1 - ((N-1)/2):1:N
    fill = zeros(size(x_tilda_k));
    fill(j,1) = sigma(j,j);
    X_Cal(:,i) = x_tilda_k - fill;
    j = j + 1;
end
end

function L = Cholesky_Decomposition(mat,method)

%% Getting size of matrix
[row,col] = size(mat);

%% Make sure matrix can be decomposed
if ~isequal(size(mat), size(mat'))
    error('Input matrix must be symmetric');
end

if any(eig(mat) <= 0)
    % error('Input matrix must be positive definite'); %% Added Error
    % Handling
    mat = NearPositiveDefinite(mat,method);
end

%% Pre allocating Space
L = zeros(row,col);

% Perform Cholesky decomposition
    for i = 1:col
        % Compute the diagonal element
        L(i, i) = sqrt(mat(i, i) - sum(L(i, 1:i-1).^2));
        
        % Compute the elements below the diagonal
        for j = i+1:col
            L(j, i) = (mat(j, i) - sum(L(j, 1:i-1).*L(i, 1:i-1))) / L(i, i);
        end
    end
end

function A_P = NearPositiveDefinite(A,method)
%% Method 1 (Symmetric Polar Factor)
%% Method 2 (Eigenvalue Recomposition)
    % enforce symmetry
    if isreal(A)
        B = 0.5*(A + A');
    else
        B = 0.5*(A + A');
        B = real(B) + 1i*hermSign(B).*imag(B);
    end

    if method == 1
        [~,~,U] = svd(B);
        H = U*U';
        A = (B + H)/2;

    elseif method == 2
        % Eigenvalue recomposition with modification for complex matrices
        [V,D] = eig(B);
        if isreal(A)
            D = max(real(D), 0); % Ensure real part of eigenvalues is non-negative
        else
            % For complex matrices, ensure positive semidefinite
            D = max(D, 0); % Ensure eigenvalues are non-negative
            V = real(V); % Take the real part of eigenvectors
        end
        A = real(V)*real(D)*real(V)'; % Now this really real product really should be really real right?
    else
        error('Please select proper method for Near Positive Definite Iteration')
    end

    % enforce symmetry again
    A_P = 0.5*(A + A');

    % Iteration
    i = 1;
    j = 0;
    max_iterations = 1000; % Maximum iterations allowed before increment starts increasing exponentially
    large_j_threshold = 500; % Threshold value for j to start increasing increment exponentially

    while i ~= 0
        [~,i] = chol(A_P);
        j = j + 1;
        if i ~= 0 % if close, add a multiple of the identity scaled by the smallest eigenvalue
            eig_min = min(eig(A_P));
            if j <= large_j_threshold
                increment = (-real(eig_min)*j.^2 + eps(real(eig_min)))*eye(size(A));
            else
                % Increase increment exponentially
                increment = (abs(real(eig_min))*j.^2 + eps(real(eig_min)))*exp(0.1*(j - large_j_threshold))*eye(size(A));
            end
            A_P = A_P + increment;
        end
        if j > max_iterations % If j exceeds the maximum allowed iterations, break the loop
            break;
        end
    end
end

function X_Cal_k1  = fcn2( F, X_Cal_k, J, m, dt)
%% Pre-Define
X_Cal_k1 = zeros(size(X_Cal_k));
%% System Dynamics
A = [eye(3), eye(3)*dt;
    zeros(3), eye(3)];

B = [eye(2)*(dt^2)/(2*m), zeros(2,1);
     0,0, (dt^2)/(2*J);
     eye(2)*(dt)/(m), zeros(2,1);
     0,0, (dt)/(J)];

%% State propigation
f = size(X_Cal_k,2);
for i = 1:1:f
    X_Cal_k1(:,i) = A*X_Cal_k(:,i) + B*F; 
end
end

function [w_m,w_c,X_tilda_k,P_K] = fcn3(X_Cal_k1,lamda, Q, alpha, beta)
%% Sigma weights
sz = size(X_Cal_k1,2);
N = 6;

%% For non modifyed variation
% w_0 = kappa/(N + kappa);
% w_i = 1/(2*(N + kappa));
% w = w_i*ones(1,N);
% w(1,1) = w_0;

%% Additional step - Sigma Points Weights
w_m_0 = lamda/(N + lamda);
w_c_0 = (lamda/(N + lamda)) + beta + (1 - alpha^2);
w_i = 1/(2*(N + lamda));

w = w_i*ones(1,sz-1);
w_m = [w_m_0, w];
w_c = [w_c_0, w];

w_m = diag(w_m);
w_c = diag(w_c);

%% State Prediction
X_tilda_k = X_Cal_k1*w_m;
X_tilda_k = sum(X_tilda_k,2);


%% Covariance Prediction
P_K = (X_Cal_k1 - X_tilda_k)*w_c*(X_Cal_k1 - X_tilda_k)' + Q;

end

function [Z_Bar,Z_Cal] = fcn4(x_Cal_k1, w_m,H)
%% calc Z_Cal
N = size(x_Cal_k1,2);
Z_Cal = zeros(3,N);
for i = 1:1:N
    Z_Cal(:,i) = H*x_Cal_k1(:,i);
end

%% Calc Z_Bar
Z_Bar = Z_Cal*w_m;
Z_Bar = sum(Z_Bar,2);
end

function [P_xz_k,P_z_k] = fcn5(Z_Bar,Z_Cal,w_c,x_tilda_k1,X_Cal,R)
%% calc P_z
P_z_k = (Z_Cal - Z_Bar)*w_c*(Z_Cal - Z_Bar)' + R;

%% calc P_xz
P_xz_k = (X_Cal - x_tilda_k1)*w_c*(Z_Cal - Z_Bar)';
end

function K_k = fcn6(P_xz_k,P_z_k)
K_k = (P_xz_k)*P_z_k';
end

function Z_k = fcn7(z_k)
    %% Assuming that all states are given or no states are given
    if anynan(z_k)
        Z_k = 1000*ones(3,1);
    else
    Z_k = z_k;
    end
end

function thresh_dynamic = Dynamic_Threshold(N_Rejectk1,thresh)
% Calculats a dynamic threshold
thresh_dynamic = thresh;
end

function  Reject = fcn8(Z_k,Z_Bar,P_z_k,thresh)
%% Calc Mahalanobis Distance
D_square = (transpose(Z_k - Z_Bar))*P_z_k*(Z_k - Z_Bar);
% mahalanobis_d = sqrt(D_square);

%% Determine if data should be rejected
if D_square < thresh
    Reject = 0;
else
    Reject = 1;
end
end

function N_Rejectk = Was_rejected(Reject,N_Rejectk1)
% Rolling average for if point was rejected
if Reject == 0
    N_Rejectk = 0;
else
    N_Rejectk = N_Rejectk1 + 1;
end
end

function [x] = fcn9(z,Reject,X_tilda_k,z_bar,K_k)
%% State estimate
    if Reject == 0
        x = X_tilda_k + K_k*(z - z_bar);
    else
        x = X_tilda_k;
    end
end

function P_K = fcn10(P_k1,P_z_k,K_k,Reject)
if Reject == 0
    P_K = P_k1 - (K_k*P_z_k)*K_k';
else
    P_K = P_k1;
end
end

== matlab function APF_Path_Planning_2023a/Phase #3: Experiment/Change RED Behavior/Sub-Phase #4/BLACK/MATLAB Function3 ==
  data: Measurments input; Black_Measurments_table_ref output; Red_States input
function Black_Measurments_table_ref = RelitivetoTable(Measurments,Red_States)
 Measurments(1) = Measurments(1)/100;
 Measurments(2) = Measurments(2)/100;
 Measurments(3) = Measurments(3)*pi/180;

%% This code is very scuffed, so I added lots of notes, feel free to change this
%% Size check
if size(Red_States,1) == 6 || size(Red_States,2) == 6
    Red_States = Red_States(1:3);
elseif size(Red_States,1) == 3 || size(Red_States,2) == 3
    % Nothin
else
    disp('Error with demensions of Red_States')
    disp('Please use 3 or 6 states')
    disp(':(')
end

if size(Measurments,1) == 3 || size(Measurments,2) == 3
    % Nothin
else
    disp('Error with demensions of Measurments')
    disp('VIS only gives 3 states, please only use 3 states')
    disp(':(')
end

%% Rotation matrix scuffed (accounts for the location change of the docking cone)
    c3 = [sin(Red_States(3)),  cos(Red_States(3)), 0;
          cos(Red_States(3)), -sin(Red_States(3)), 0;
          0,                     0,                    1];

%% Measurments in table ref frame
    Black_Measurments_table_ref = c3*Measurments;

%% Vector addition
    Black_Measurments_table_ref(1) = Black_Measurments_table_ref(1) + Red_States(1); 
    Black_Measurments_table_ref(2) =  -1*Black_Measurments_table_ref(2) + Red_States(2); % Negative Y value accounting for "Left Hand Rule"

%% Angle addition
    Black_Measurments_table_ref(3) = Measurments(3) + Red_States(3) - pi/2; % Pi/2 for the docking cone location offset from Phase Space

%% Wrapping Angle from -pi to pi
% Dont ask me why, its consistant with the SPOT inport from phasespace
% Dont belive me, look at this, angular velocity is being unwrapped, therefor, angle must be wrapped
% APF_Path_Planning_2023a/PhaseSpace Camera Code/Use Hardware to Obtain States
    Black_Measurments_table_ref(3) = mod(Black_Measurments_table_ref(3) + pi, 2*pi) - pi;
end

== matlab function APF_Path_Planning_2023a/Phase #5: Hold Home/Change BLUE Behavior/Hough Control/MATLAB Function2 ==
  data: Oy output; z input; Ox output
function [Oy, Ox]   = C3( z )
%C3 gives the rotation matrix about the z-axis for an angle 'z'
%   z - the angle about the z-axis which you rotate
%   A - the rotation matrix

Ox = [cos(z) sin(z); -sin(z) cos(z)]*[1;0];
Oy = [cos(z) sin(z); -sin(z) cos(z)]*[0;1];
end

== matlab function APF_Path_Planning_2023a/Phase #3: Experiment/Change RED Behavior/Sub-Phase #4/GDC/Target Tracker/Constant Angular Rate/Looking Angle ==
  data: state_black input; state_red input; theta_desired output; r_off parameter
function theta_desired = fcn(state_black, state_red, r_off)

p_l = [state_black(1) + r_off*cos(state_black(3));
       state_black(2) + r_off*sin(state_black(3))];

p_c_1 = state_red(1:2);
r_cl = p_c_1 - p_l;

r_cl_x = r_cl(1);
r_cl_y = r_cl(2);

theta_desired = angle(r_cl_x + 1j*r_cl_y) + pi;

== matlab function APF_Path_Planning_2023a/Phase #3: Experiment/Change RED Behavior/Sub-Phase #4/CTL/Target Finder/LQR1/MATLAB Function ==
  data: k input; u output; q1_x input; q2_x input; q1_y input; q2_y input; q1_t input; q2_t input
function u = fcn(k,q1_x,q2_x,q1_y,q2_y,q1_t,q2_t)

x = [q1_x;
    q1_y;
    q1_t;
    q2_x;
    q2_y;
    q2_t];

u = k*x;
% u = [0; 0; 0];

== matlab function APF_Path_Planning_2023a/Phase #3: Experiment/Change BLUE Behavior/Sub-Phase #2 /MATLAB Function2 ==
  data: t input; x output; xLength parameter
function x = fcn(t, xLength)

x = -0.85*cos((0.03490659)*t) + xLength/2;

end

== matlab function APF_Path_Planning_2023a/Phase #3: Experiment/Change BLUE Behavior/Sub-Phase #2 /MATLAB Function3 ==
  data: t input; y output; yLength parameter
function y = fcn(t, yLength)

y = -0.85*sin((0.03490659)*t) + yLength/2;

end

== matlab function APF_Path_Planning_2023a/Phase #3: Experiment/Change RED Behavior/Sub-Phase #4/BLACK/MEKF/MATLAB Function ==
  data: Measurments input; States output; F input; X_tilda_k input; P_k1 input; P_K output; J parameter; m parameter; dt parameter; Q parameter; R parameter; H parameter; thresh parameter
function [States, P_K]  = MEKF(Measurments,F,X_tilda_k,P_k1, J, m, dt, Q, R, H, thresh)

if isempty(F)
    F = [0;0;0];
end

    %% Body
    [x_tilda_k1,P_k1] = fcn1( F, m, J, dt, X_tilda_k, P_k1,Q);
    
    K_k = fcn2(P_k1,R, H);

    Z_k = fcn7(Measurments);
    
    Y_k = fcn3(Z_k,H,x_tilda_k1);
    
    [~, Reject] = fnc4(Z_k, x_tilda_k1, P_k1,thresh,H);
    
    States = fcn5(Y_k,X_tilda_k,Reject,K_k);
    
    P_K = fcn(P_k1,K_k,H);
end

function [x_tilda_k1,P_k1] = fcn1( F, m, J, dt, X_tilda_k, P_k,Q)

A = [eye(3), eye(3)*dt;
    zeros(3), eye(3)];

G = [eye(2)*(dt^2)/(2*m), zeros(2,4);
     zeros(1,2), (dt^2)/(2*J), zeros(1,3);
     zeros(2,4), eye(2)*(dt)/(m);
     zeros(1,5), (dt)/(J)];
B = [eye(2)*(dt^2)/(2*m), zeros(2,1);
     0,0, (dt^2)/(2*J);
     eye(2)*(dt)/(m),zeros(2,1);
     0,0, (dt)/(J)];

x_tilda_k1 = A*X_tilda_k + B*F; %State prediction
P_k1 = A'*P_k*A;
P_k1 = P_k1 + G'*Q*G; %covariance predict
P_k1 = 0.5*(P_k1 + P_k1'); %enforce symmetric
end

function K_k = fcn2(P_k1,R, H)
Sk = H*P_k1*H' + R;
K_k = P_k1*H'*inv(Sk);
end

function Z_k = fcn7(z_k)
    %% Assuming that all states are given or no states are given
    if anynan(z_k)
        Z_k = 1000*ones(3,1);
    else
    Z_k = z_k;
    end
end

function Y_k = fcn3(Z_k,H,X_tilda_k1)
Y_k = Z_k - H*X_tilda_k1;
end

function [mahalanobis_d, Reject] = fnc4(z_k, X_tilda_k1, Pk1,thresh,H)
    % measurement: Measurement vector
    % stateEstimate: Estimated state vector (6x1)
    % covarianceMatrix: Covariance matrix of the state estimate (6x6)

    % Number of state variables
    numVariables = length(X_tilda_k1);

    % Residual vector
    residual = z_k - H*X_tilda_k1;

    % Mahalanobis distance calculation
    mahalanobis_d = sqrt(residual' * inv(Pk1(1:3,1:3)) * residual);
    threshold = thresh;

    % If Mahalanobis distance exceeds the threshold, consider it an outlier
    if mahalanobis_d > threshold
        Reject = 1;
    else
        Reject = 0;
    end
end

function x = fcn5(Y_k,X_tilda_k,Reject,K_k)
    if Reject == 0
        x = X_tilda_k + K_k*Y_k;
    else
        x = X_tilda_k;
    end
end

function P_K = fcn(P_k1,K_k,H)
P_K = zeros(6,6);
P_K = (eye(6) - K_k*H)*P_k1*transpose(eye(6) - K_k*H) + K_k*K_k'; 
P_k = 0.5*(P_K'+P_K); % make covariance matrix symmetric
end

== matlab function APF_Path_Planning_2023a/Thruster Control Code/Change BLUE Behavior/Calculate Thruster ON//OFF/MATLAB Function6 ==
  data: thrust_decay_factor output; PWMs input; thruster_count_threshold parameter; count output
function [thrust_decay_factor, count]  = check_thrust_decay(PWMs,thruster_count_threshold)

% normalize PWMs
if max(PWMs) > 1
    PWMs = PWMs/max(PWMs);
end

count = sum(PWMs > thruster_count_threshold);

positives_only = max(PWMs,0);
sum_of_duty_cycles = sum(positives_only);

average_duty_cycle_per_thruster = sum_of_duty_cycles/count;

% Look up the thrust decay for this average duty cycle
if (average_duty_cycle_per_thruster < 0.3) || (count == 0)
    thrust_decay_factor = 1;
else
    thrust_decay_factor = max(0.6 - 2*average_duty_cycle_per_thruster + 1, 0.5);   
end

== matlab function APF_Path_Planning_2023a/Thruster Control Code/Change BLUE Behavior/Calculate Thruster ON//OFF/MATLAB Function7 ==
  data: H output; thruster_dist2CG_BLUE parameter; F_Blue_X_nominal parameter; thrust_decay_factor input; F_Blue_Y_nominal parameter
function H   = MakeHWithDecay(thruster_dist2CG_BLUE,F_Blue_X_nominal, thrust_decay_factor, F_Blue_Y_nominal)


adjusted_thruster_dist2CG_BLUE = [thruster_dist2CG_BLUE(1);
                                 thruster_dist2CG_BLUE(2);
                                 thruster_dist2CG_BLUE(3);
                                 thruster_dist2CG_BLUE(4);
                                 thruster_dist2CG_BLUE(5);
                                 thruster_dist2CG_BLUE(6);
                                 thruster_dist2CG_BLUE(7);
                                 thruster_dist2CG_BLUE(8)];
                                 


Vec1 = [ -1
         -1
          0 
          0
          1
          1
          0
          0 ];
      
Vec2 = [  0
          0
          1
          1
          0
          0
         -1
         -1 ];
     
Vec3 = adjusted_thruster_dist2CG_BLUE./1000;

Mat1 = [Vec1, Vec2, Vec3]';

F_thrusters_BLUE = [F_Blue_X_nominal*thrust_decay_factor; F_Blue_X_nominal*thrust_decay_factor; F_Blue_Y_nominal*thrust_decay_factor; F_Blue_Y_nominal*thrust_decay_factor; F_Blue_X_nominal*thrust_decay_factor; F_Blue_X_nominal*thrust_decay_factor; F_Blue_Y_nominal*thrust_decay_factor; F_Blue_Y_nominal*thrust_decay_factor];

Mat2 = diag((F_thrusters_BLUE./2));

H    = Mat1*Mat2;

end

== matlab function APF_Path_Planning_2023a/Thruster Control Code/Change BLACK Behavior/Calculate Thruster ON//OFF/MATLAB Function10 ==
  data: thrust_decay_factor output; PWMs input; thruster_count_threshold parameter; count output
function [thrust_decay_factor, count]  = check_thrust_decay(PWMs,thruster_count_threshold)

% normalize PWMs
if max(PWMs) > 1
    PWMs = PWMs/max(PWMs);
end

count = sum(PWMs > thruster_count_threshold);

positives_only = max(PWMs,0);
sum_of_duty_cycles = sum(positives_only);

average_duty_cycle_per_thruster = sum_of_duty_cycles/count;

% Look up the thrust decay for this average duty cycle
if (average_duty_cycle_per_thruster < 0.3) || (count == 0)
    thrust_decay_factor = 1;
else
    thrust_decay_factor = max(0.6 - 2*average_duty_cycle_per_thruster + 1, 0.5);   
end

== matlab function APF_Path_Planning_2023a/Phase #5: Hold Home/Change BLUE Behavior/Hough Control/MATLAB Function3 ==
  data: z input; Ox output
function Ox    = C3( z )
%C3 gives the rotation matrix about the z-axis for an angle 'z'
%   z - the angle about the z-axis which you rotate
%   A - the rotation matrix

Ox = [cos(z) sin(z); -sin(z) cos(z)]*[1;0];
end

== matlab function APF_Path_Planning_2023a/Thruster Control Code/Change BLACK Behavior/Calculate Thruster ON//OFF/MATLAB Function11 ==
  data: H output; thruster_dist2CG_BLACK parameter; F_Black_X_nominal parameter; thrust_decay_factor input; F_Black_Y_nominal parameter
function H   = MakeHWithDecay(thruster_dist2CG_BLACK,F_Black_X_nominal, thrust_decay_factor, F_Black_Y_nominal)


adjusted_thruster_dist2CG_BLACK = [thruster_dist2CG_BLACK(1);
                                 thruster_dist2CG_BLACK(2);
                                 thruster_dist2CG_BLACK(3);
                                 thruster_dist2CG_BLACK(4);
                                 thruster_dist2CG_BLACK(5);
                                 thruster_dist2CG_BLACK(6);
                                 thruster_dist2CG_BLACK(7);
                                 thruster_dist2CG_BLACK(8)];
                                 


Vec1 = [ -1
         -1
          0 
          0
          1
          1
          0
          0 ];
      
Vec2 = [  0
          0
          1
          1
          0
          0
         -1
         -1 ];
     
Vec3 = adjusted_thruster_dist2CG_BLACK./1000;

Mat1 = [Vec1, Vec2, Vec3]';

F_thrusters_BLACK = [F_Black_X_nominal*thrust_decay_factor; F_Black_X_nominal*thrust_decay_factor; F_Black_Y_nominal*thrust_decay_factor; F_Black_Y_nominal*thrust_decay_factor; F_Black_X_nominal*thrust_decay_factor; F_Black_X_nominal*thrust_decay_factor; F_Black_Y_nominal*thrust_decay_factor; F_Black_Y_nominal*thrust_decay_factor];

Mat2 = diag((F_thrusters_BLACK./2));

H    = Mat1*Mat2;

end
